simulink model "Example_OB_Dynamic_Undirected_LeaderFollower"  (R2023b)
settings: Solver=FixedStepAuto  StartTime=0.0  StopTime=20  FixedStep=0.001  RelTol=1e-3  EnableMultiTasking=on
values from neighbouring files (symbols this model uses):
  A = [0  1  0 ... (first row only)    [Code_OB_Dynamic_Undirected_LeaderFollower.m]
  ADJ = [0  1  1  0  0  0  0 ... (first row only)    [Code_OB_Dynamic_Undirected_LeaderFollower.m]
  BB = [1  0  1  0  0  1  0]*0    [Code_OB_Dynamic_Undirected_LeaderFollower.m]
  Bu = [0;0;1]    [Code_OB_Dynamic_Undirected_LeaderFollower.m]
  c = 1/lambda1    [Code_OB_Dynamic_Undirected_LeaderFollower.m]
  Cy = [1 0 0]    [Code_OB_Dynamic_Undirected_LeaderFollower.m]
  delta = 0.9*min(min(abs(eig(Q)))/max(abs(eig(P))),min(alpha))    [Code_OB_Dynamic_Undirected_LeaderFollower.m]
  eta1 = 1    [Code_OB_Dynamic_Undirected_LeaderFollower.m]
  eta2 = 1    [Code_OB_Dynamic_Undirected_LeaderFollower.m]
  eta3 = 1    [Code_OB_Dynamic_Undirected_LeaderFollower.m]
  eta4 = 1    [Code_OB_Dynamic_Undirected_LeaderFollower.m]
  eta5 = 1    [Code_OB_Dynamic_Undirected_LeaderFollower.m]
  eta6 = 1    [Code_OB_Dynamic_Undirected_LeaderFollower.m]
  F = -P*Cy'    [Code_OB_Dynamic_Undirected_LeaderFollower.m]
  K = -Bu'*P    [Code_OB_Dynamic_Undirected_LeaderFollower.m]
  kappa = 0.1    [Code_OB_Dynamic_Undirected_LeaderFollower.m]
  LL = diag(sum(ADJ,2))-ADJ    [Code_OB_Dynamic_Undirected_LeaderFollower.m]
  mu = 0.5    [Code_OB_Dynamic_Undirected_LeaderFollower.m]
  N = length(LL)    [Code_OB_Dynamic_Undirected_LeaderFollower.m]
  nr = nx    [Code_OB_Dynamic_Undirected_LeaderFollower.m]
  nx = size(A,1)    [Code_OB_Dynamic_Undirected_LeaderFollower.m]
  ny = size(Cy,1)    [Code_OB_Dynamic_Undirected_LeaderFollower.m]
  Tc = linspace(0.1,0.7,7)    [Code_OB_Dynamic_Undirected_LeaderFollower.m]
  Th = 10    [Code_OB_Dynamic_Undirected_LeaderFollower.m]
  x0 = x_leader.Data    [Code_OB_Dynamic_Undirected_LeaderFollower.m]
  x0_leader = [1 1 1]    [Code_OB_Dynamic_Undirected_LeaderFollower.m]
undefined symbols (not defined in the file or in its folder): Kri_m_Krj_1, Kri_m_Krj_2, Kri_m_Krj_3, Kri_m_Krj_4, Kri_m_Krj_5, Kri_m_Krj_6, Kri_m_Krj_7, ty0_1, ty0_2, ty0_3, ty0_4, ty0_5, ty0_6, ty0_7
settings Model: PauseTimes=0.9999  Creator=Xianwei  LastModifiedBy=30970
settings SolverCC: AlgebraicLoopSolver=LineSearch
settings DataIOCC: LimitDataPoints=on  ReturnWorkspaceOutputs=off
settings OptimizationCC: LifeSpan=inf
settings DebuggingCC: UnconnectedInputMsg=warning  UnconnectedOutputMsg=warning  UnconnectedLineMsg=warning  AllowSymbolicDim=off  SFUnexpectedBacktrackingDiag=warning  SFNoUnconditionalDefaultTransitionDiag=warning  SFExecutionAtInitializationDiag=none  ArithmeticOperatorsInVariantConditions=warning
settings ModelReferenceCC: EnableRefExpFcnMdlSchedulingChecks=on  PropagateSignalLabelsOutOfModel=off
settings SFSimCC: SimUseLocalCustomCode=off  CustomCodeUndefinedFunction=UseInterfaceOnly
settings RTWCC: RTWUseLocalCustomCode=off  DLArmComputeVersion=19.05
settings CodeAppCC: StateflowObjectComments=on
settings GRTTargetCC: TargetLangStandard=C89/C90 (ANSI)
settings ConfigComp: CovMetricSettings=dw  CovSaveCumulativeToWorkspaceVar=on  CovSaveSingleToWorkspaceVar=on  CovExternalEMLEnable=off

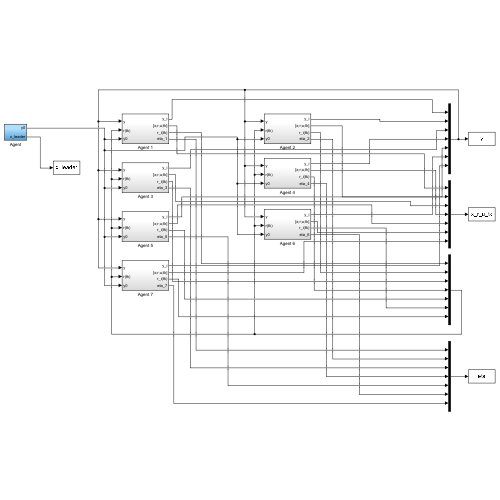
[thumbnail: Simulink's stored preview of the top-level diagram]
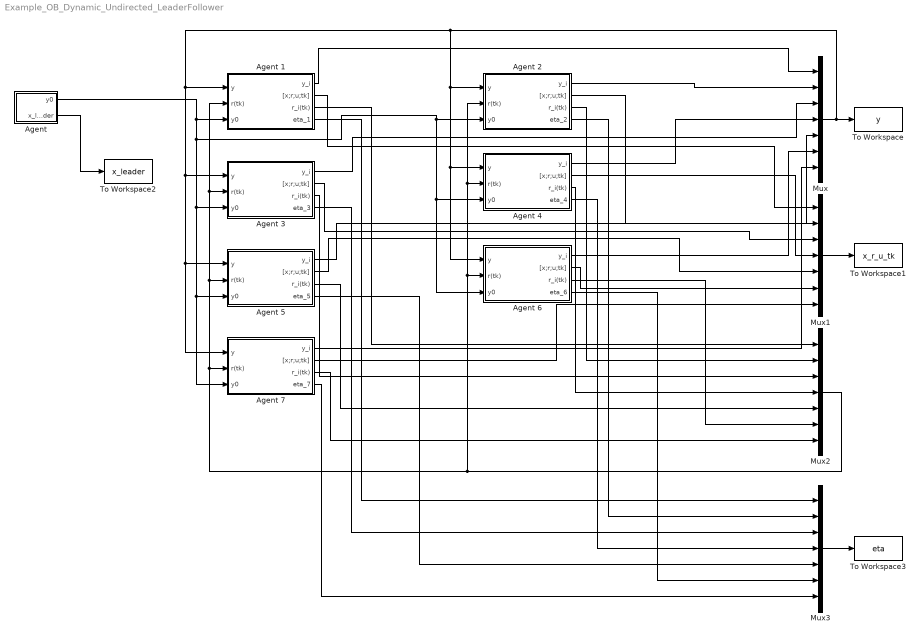
== system Example_OB_Dynamic_Undirected_LeaderFollower ==
  Agent : Subsystem
  Agent 1 : Subsystem
  Agent 2 : Subsystem
  Agent 3 : Subsystem
  Agent 4 : Subsystem
  Agent 5 : Subsystem
  Agent 6 : Subsystem
  Agent 7 : Subsystem
  Mux{,1..3} (4 alike) : Mux  Inputs=7
  To Workspace : ToWorkspace  VariableName=y  SaveFormat=Timeseries  SampleTime=-1
  To Workspace1 : ToWorkspace  VariableName=x_r_u_tk  SaveFormat=Timeseries  SampleTime=-1
  To Workspace2 : ToWorkspace  VariableName=x_leader  SaveFormat=Timeseries  SampleTime=-1
  To Workspace3 : ToWorkspace  VariableName=eta  SaveFormat=Timeseries  SampleTime=-1
  wires:
  Mux1/1 -> To Workspace1/1
  Agent 1/1(y_i) -> Mux/1
  Agent 2/1(y_i) -> Mux/2
  Agent 3/1(y_i) -> Mux/3
  Agent 4/1(y_i) -> Mux/4
  Agent 5/1(y_i) -> Mux/5
  Agent 1/2("[x;r;u;tk]") -> Mux1/1
  Agent 2/2("[x;r;u;tk]") -> Mux1/2
  Agent 3/2("[x;r;u;tk]") -> Mux1/3
  Agent 4/2("[x;r;u;tk]") -> Mux1/4
  Agent 5/2("[x;r;u;tk]") -> Mux1/5
  Agent 1/3(r_i(tk)) -> Mux2/1
  Agent 2/3(r_i(tk)) -> Mux2/2
  Agent 3/3(r_i(tk)) -> Mux2/3
  Agent 4/3(r_i(tk)) -> Mux2/4
  Agent 5/3(r_i(tk)) -> Mux2/5
  Agent 6/3(r_i(tk)) -> Mux2/6
  Agent 6/1(y_i) -> Mux/6
  Agent 6/2("[x;r;u;tk]") -> Mux1/6
  Agent 7/1(y_i) -> Mux/7
  Agent 7/2("[x;r;u;tk]") -> Mux1/7
  Agent 7/3(r_i(tk)) -> Mux2/7
  Mux/1 -> Agent 7/1(y), Agent 5/1(y), Agent 3/1(y), Agent 1/1(y), Agent 6/1(y), Agent 4/1(y), Agent 2/1(y), To Workspace/1
  Mux2/1 -> Agent 1/2(r(tk)), Agent 3/2(r(tk)), Agent 5/2(r(tk)), Agent 7/2(r(tk)), Agent 2/2(r(tk)), Agent 4/2(r(tk)), Agent 6/2(r(tk))
  Agent/1(y0) -> Agent 6/3(y0), Agent 4/3(y0), Agent 2/3(y0), Agent 7/3(y0), Agent 5/3(y0), Agent 3/3(y0), Agent 1/3(y0)
  Agent/2(x_leader) -> To Workspace2/1
  Agent 1/4(eta_1) -> Mux3/1
  Mux3/1 -> To Workspace3/1
  Agent 2/4(eta_2) -> Mux3/2
  Agent 3/4(eta_3) -> Mux3/3
  Agent 4/4(eta_4) -> Mux3/4
  Agent 5/4(eta_5) -> Mux3/5
  Agent 6/4(eta_6) -> Mux3/6
  Agent 7/4(eta_7) -> Mux3/7

== system Example_OB_Dynamic_Undirected_LeaderFollower/Agent ==
  A : Gain  Gain=A  Multiplication=Matrix(K*u)
  Cy : Gain  Gain=Cy  Multiplication=Matrix(K*u)
  Integrator : Integrator  InitialCondition=x0_leader  ContinuousStateAttributes='x1'
  y0 : Outport
  x_leader : Outport  Port=2
  wires:
  Integrator/1 -> x_leader/1, A/1, Cy/1
  A/1 -> Integrator/1
  Cy/1 -> y0/1

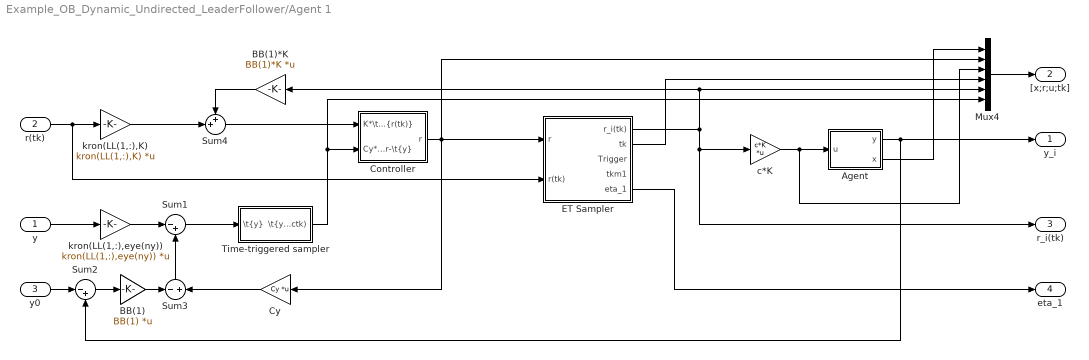
== system Example_OB_Dynamic_Undirected_LeaderFollower/Agent 1 ==
  y : Inport
  r(tk) : Inport  Port=2
  y0 : Inport  Port=3
  Agent : Subsystem
  BB(1) : Gain  Gain=BB(1)  Multiplication=Matrix(K*u)
  BB(1)*K : Gain  Gain=BB(1)*K  Multiplication=Matrix(K*u)
  Controller : Subsystem
  Cy : Gain  Gain=Cy  Multiplication=Matrix(K*u)
  ET Sampler : Subsystem
  Mux4 : Mux  Inputs=6
  Sum1 : Sum  Inputs=|-+
  Sum2 : Sum  Inputs=|-+
  Sum3 : Sum  Inputs=-|+
  Sum4 : Sum  Inputs=++|
  Time-triggered sampler : Subsystem
  c*K : Gain  Gain=c*K  Multiplication=Matrix(K*u)
  kron(LL(1,:),K) : Gain  Gain=kron(LL(1,:),K)  Multiplication=Matrix(K*u)
  kron(LL(1,:),eye(ny)) : Gain  Gain=kron(LL(1,:),eye(ny))  Multiplication=Matrix(K*u)
  y_i : Outport
  "[x;r;u;tk]" : Outport  Port=2
  r_i(tk) : Outport  Port=3
  eta_1 : Outport  Port=4
  wires:
  Agent/2(x) -> Mux4/1
  Mux4/1 -> "[x;r;u;tk]"/1
  ET Sampler/2(tk) -> Mux4/4
  c*K/1 -> Agent/1(u), Mux4/3
  y/1 -> kron(LL(1,:),eye(ny))/1
  r(tk)/1 -> kron(LL(1,:),K)/1, ET Sampler/2(r(tk))
  kron(LL(1,:),K)/1 -> Sum4/2
  ET Sampler/1(r_i(tk)) -> BB(1)*K/1, Mux4/5, c*K/1, r_i(tk)/1
  Controller/1(r) -> Cy/1, ET Sampler/1(r), Mux4/2
  Cy/1 -> Sum3/2
  Sum1/1 -> Time-triggered sampler/1("\\t{y}")
  kron(LL(1,:),eye(ny))/1 -> Sum1/1
  Time-triggered sampler/1("\\t{y}(ctk)") -> Mux4/6, Controller/2("Cy*r-\\t{y}")
  y0/1 -> Sum2/1
  Agent/1(y) -> Sum2/2, y_i/1
  Sum2/1 -> BB(1)/1
  BB(1)/1 -> Sum3/1
  Sum3/1 -> Sum1/2
  BB(1)*K/1 -> Sum4/1
  Sum4/1 -> Controller/1("K*\\t{r(tk)}")
  ET Sampler/5(eta_1) -> eta_1/1

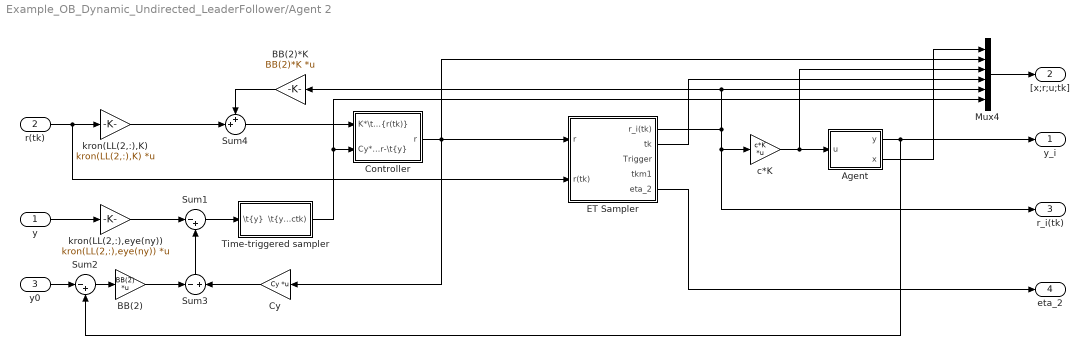
== system Example_OB_Dynamic_Undirected_LeaderFollower/Agent 2 ==
  y : Inport
  r(tk) : Inport  Port=2
  y0 : Inport  Port=3
  Agent : Subsystem
  BB(2) : Gain  Gain=BB(2)  Multiplication=Matrix(K*u)
  BB(2)*K : Gain  Gain=BB(2)*K  Multiplication=Matrix(K*u)
  Controller : Subsystem
  Cy : Gain  Gain=Cy  Multiplication=Matrix(K*u)
  ET Sampler : Subsystem
  Mux4 : Mux  Inputs=6
  Sum1 : Sum  Inputs=|-+
  Sum2 : Sum  Inputs=|-+
  Sum3 : Sum  Inputs=-|+
  Sum4 : Sum  Inputs=++|
  Time-triggered sampler : Subsystem
  c*K : Gain  Gain=c*K  Multiplication=Matrix(K*u)
  kron(LL(2,:),K) : Gain  Gain=kron(LL(2,:),K)  Multiplication=Matrix(K*u)
  kron(LL(2,:),eye(ny)) : Gain  Gain=kron(LL(2,:),eye(ny))  Multiplication=Matrix(K*u)
  y_i : Outport
  "[x;r;u;tk]" : Outport  Port=2
  r_i(tk) : Outport  Port=3
  eta_2 : Outport  Port=4
  wires:
  c*K/1 -> Agent/1(u), Mux4/3
  r(tk)/1 -> ET Sampler/2(r(tk)), kron(LL(2,:),K)/1
  kron(LL(2,:),K)/1 -> Sum4/2
  Mux4/1 -> "[x;r;u;tk]"/1
  Controller/1(r) -> ET Sampler/1(r), Mux4/2, Cy/1
  Agent/2(x) -> Mux4/1
  kron(LL(2,:),eye(ny))/1 -> Sum1/1
  ET Sampler/2(tk) -> Mux4/4
  y/1 -> kron(LL(2,:),eye(ny))/1
  Cy/1 -> Sum3/2
  Sum1/1 -> Time-triggered sampler/1("\\t{y}")
  Time-triggered sampler/1("\\t{y}(ctk)") -> Mux4/6, Controller/2("Cy*r-\\t{y}")
  y0/1 -> Sum2/1
  Agent/1(y) -> Sum2/2, y_i/1
  BB(2)/1 -> Sum3/1
  Sum2/1 -> BB(2)/1
  Sum3/1 -> Sum1/2
  BB(2)*K/1 -> Sum4/1
  ET Sampler/1(r_i(tk)) -> BB(2)*K/1, Mux4/5, r_i(tk)/1, c*K/1
  Sum4/1 -> Controller/1("K*\\t{r(tk)}")
  ET Sampler/5(eta_2) -> eta_2/1

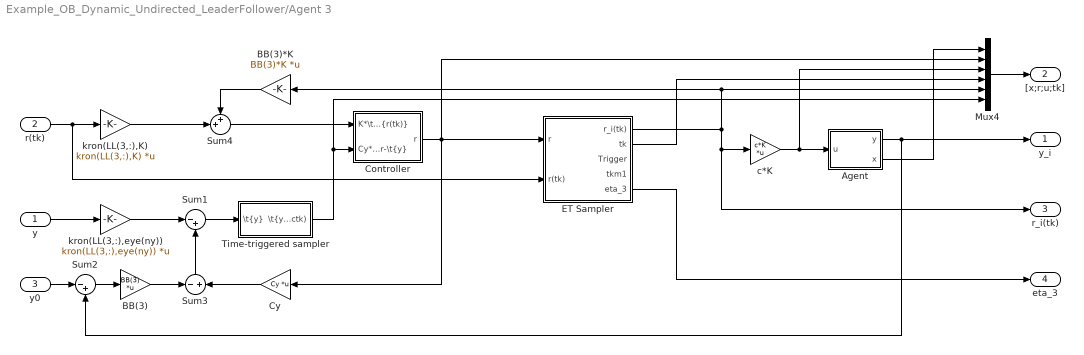
== system Example_OB_Dynamic_Undirected_LeaderFollower/Agent 3 ==
  y : Inport
  r(tk) : Inport  Port=2
  y0 : Inport  Port=3
  Agent : Subsystem
  BB(3) : Gain  Gain=BB(3)  Multiplication=Matrix(K*u)
  BB(3)*K : Gain  Gain=BB(3)*K  Multiplication=Matrix(K*u)
  Controller : Subsystem
  Cy : Gain  Gain=Cy  Multiplication=Matrix(K*u)
  ET Sampler : Subsystem
  Mux4 : Mux  Inputs=6
  Sum1 : Sum  Inputs=|-+
  Sum2 : Sum  Inputs=|-+
  Sum3 : Sum  Inputs=-|+
  Sum4 : Sum  Inputs=++|
  Time-triggered sampler : Subsystem
  c*K : Gain  Gain=c*K  Multiplication=Matrix(K*u)
  kron(LL(3,:),K) : Gain  Gain=kron(LL(3,:),K)  Multiplication=Matrix(K*u)
  kron(LL(3,:),eye(ny)) : Gain  Gain=kron(LL(3,:),eye(ny))  Multiplication=Matrix(K*u)
  y_i : Outport
  "[x;r;u;tk]" : Outport  Port=2
  r_i(tk) : Outport  Port=3
  eta_3 : Outport  Port=4
  wires:
  c*K/1 -> Agent/1(u), Mux4/3
  r(tk)/1 -> ET Sampler/2(r(tk)), kron(LL(3,:),K)/1
  kron(LL(3,:),K)/1 -> Sum4/2
  Mux4/1 -> "[x;r;u;tk]"/1
  Controller/1(r) -> ET Sampler/1(r), Mux4/2, Cy/1
  Agent/2(x) -> Mux4/1
  kron(LL(3,:),eye(ny))/1 -> Sum1/1
  ET Sampler/2(tk) -> Mux4/4
  y/1 -> kron(LL(3,:),eye(ny))/1
  Cy/1 -> Sum3/2
  Sum1/1 -> Time-triggered sampler/1("\\t{y}")
  Time-triggered sampler/1("\\t{y}(ctk)") -> Mux4/6, Controller/2("Cy*r-\\t{y}")
  Sum2/1 -> BB(3)/1
  BB(3)/1 -> Sum3/1
  Agent/1(y) -> Sum2/2, y_i/1
  y0/1 -> Sum2/1
  Sum3/1 -> Sum1/2
  BB(3)*K/1 -> Sum4/1
  ET Sampler/1(r_i(tk)) -> BB(3)*K/1, Mux4/5, r_i(tk)/1, c*K/1
  Sum4/1 -> Controller/1("K*\\t{r(tk)}")
  ET Sampler/5(eta_3) -> eta_3/1

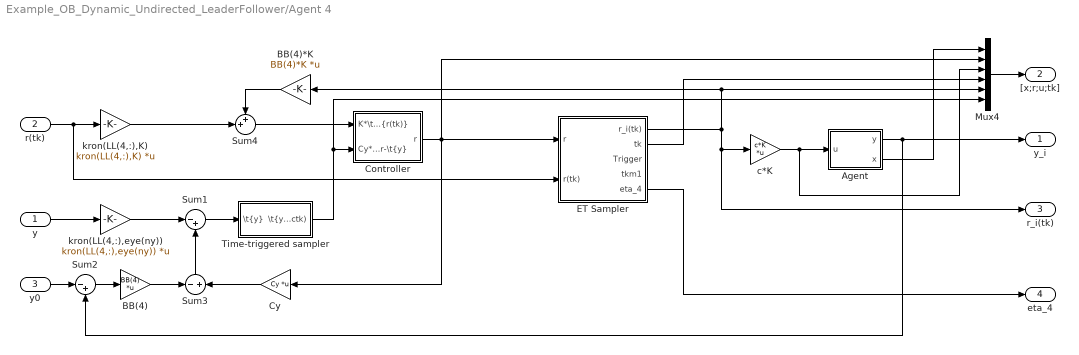
== system Example_OB_Dynamic_Undirected_LeaderFollower/Agent 4 ==
  y : Inport
  r(tk) : Inport  Port=2
  y0 : Inport  Port=3
  Agent : Subsystem
  BB(4) : Gain  Gain=BB(4)  Multiplication=Matrix(K*u)
  BB(4)*K : Gain  Gain=BB(4)*K  Multiplication=Matrix(K*u)
  Controller : Subsystem
  Cy : Gain  Gain=Cy  Multiplication=Matrix(K*u)
  ET Sampler : Subsystem
  Mux4 : Mux  Inputs=6
  Sum1 : Sum  Inputs=|-+
  Sum2 : Sum  Inputs=|-+
  Sum3 : Sum  Inputs=-|+
  Sum4 : Sum  Inputs=++|
  Time-triggered sampler : Subsystem
  c*K : Gain  Gain=c*K  Multiplication=Matrix(K*u)
  kron(LL(4,:),K) : Gain  Gain=kron(LL(4,:),K)  Multiplication=Matrix(K*u)
  kron(LL(4,:),eye(ny)) : Gain  Gain=kron(LL(4,:),eye(ny))  Multiplication=Matrix(K*u)
  y_i : Outport
  "[x;r;u;tk]" : Outport  Port=2
  r_i(tk) : Outport  Port=3
  eta_4 : Outport  Port=4
  wires:
  y/1 -> kron(LL(4,:),eye(ny))/1
  Sum1/1 -> Time-triggered sampler/1("\\t{y}")
  Mux4/1 -> "[x;r;u;tk]"/1
  c*K/1 -> Agent/1(u), Mux4/3
  ET Sampler/2(tk) -> Mux4/4
  r(tk)/1 -> ET Sampler/2(r(tk)), kron(LL(4,:),K)/1
  Controller/1(r) -> ET Sampler/1(r), Mux4/2, Cy/1
  Agent/2(x) -> Mux4/1
  kron(LL(4,:),K)/1 -> Sum4/2
  kron(LL(4,:),eye(ny))/1 -> Sum1/1
  Time-triggered sampler/1("\\t{y}(ctk)") -> Mux4/6, Controller/2("Cy*r-\\t{y}")
  Sum2/1 -> BB(4)/1
  BB(4)/1 -> Sum3/1
  Agent/1(y) -> Sum2/2, y_i/1
  y0/1 -> Sum2/1
  Sum3/1 -> Sum1/2
  Cy/1 -> Sum3/2
  BB(4)*K/1 -> Sum4/1
  ET Sampler/1(r_i(tk)) -> BB(4)*K/1, Mux4/5, r_i(tk)/1, c*K/1
  Sum4/1 -> Controller/1("K*\\t{r(tk)}")
  ET Sampler/5(eta_4) -> eta_4/1

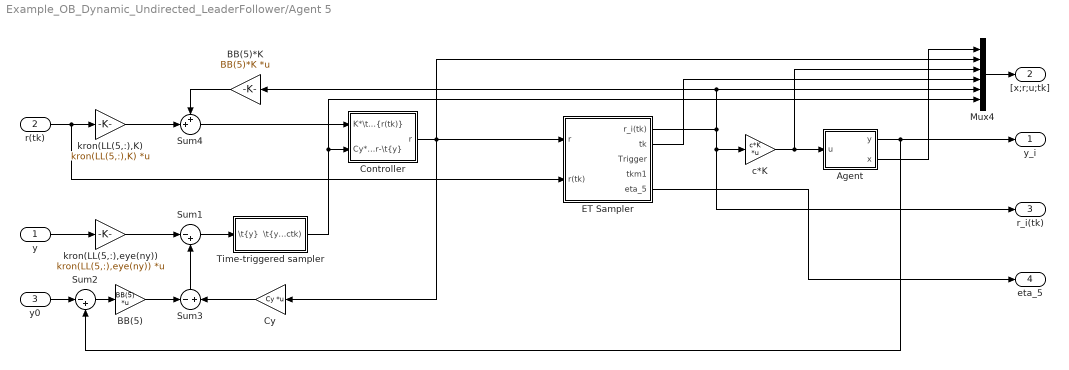
== system Example_OB_Dynamic_Undirected_LeaderFollower/Agent 5 ==
  y : Inport
  r(tk) : Inport  Port=2
  y0 : Inport  Port=3
  Agent : Subsystem
  BB(5) : Gain  Gain=BB(5)  Multiplication=Matrix(K*u)
  BB(5)*K : Gain  Gain=BB(5)*K  Multiplication=Matrix(K*u)
  Controller : Subsystem
  Cy : Gain  Gain=Cy  Multiplication=Matrix(K*u)
  ET Sampler : Subsystem
  Mux4 : Mux  Inputs=6
  Sum1 : Sum  Inputs=|-+
  Sum2 : Sum  Inputs=|-+
  Sum3 : Sum  Inputs=-|+
  Sum4 : Sum  Inputs=++|
  Time-triggered sampler : Subsystem
  c*K : Gain  Gain=c*K  Multiplication=Matrix(K*u)
  kron(LL(5,:),K) : Gain  Gain=kron(LL(5,:),K)  Multiplication=Matrix(K*u)
  kron(LL(5,:),eye(ny)) : Gain  Gain=kron(LL(5,:),eye(ny))  Multiplication=Matrix(K*u)
  y_i : Outport
  "[x;r;u;tk]" : Outport  Port=2
  r_i(tk) : Outport  Port=3
  eta_5 : Outport  Port=4
  wires:
  kron(LL(5,:),eye(ny))/1 -> Sum1/1
  kron(LL(5,:),K)/1 -> Sum4/2
  Agent/2(x) -> Mux4/1
  Controller/1(r) -> ET Sampler/1(r), Mux4/2, Cy/1
  ET Sampler/2(tk) -> Mux4/4
  Sum1/1 -> Time-triggered sampler/1("\\t{y}")
  c*K/1 -> Agent/1(u), Mux4/3
  Mux4/1 -> "[x;r;u;tk]"/1
  r(tk)/1 -> ET Sampler/2(r(tk)), kron(LL(5,:),K)/1
  y/1 -> kron(LL(5,:),eye(ny))/1
  Time-triggered sampler/1("\\t{y}(ctk)") -> Mux4/6, Controller/2("Cy*r-\\t{y}")
  Sum2/1 -> BB(5)/1
  BB(5)/1 -> Sum3/1
  Agent/1(y) -> Sum2/2, y_i/1
  y0/1 -> Sum2/1
  Cy/1 -> Sum3/2
  Sum3/1 -> Sum1/2
  BB(5)*K/1 -> Sum4/1
  ET Sampler/1(r_i(tk)) -> Mux4/5, BB(5)*K/1, r_i(tk)/1, c*K/1
  Sum4/1 -> Controller/1("K*\\t{r(tk)}")
  ET Sampler/5(eta_5) -> eta_5/1

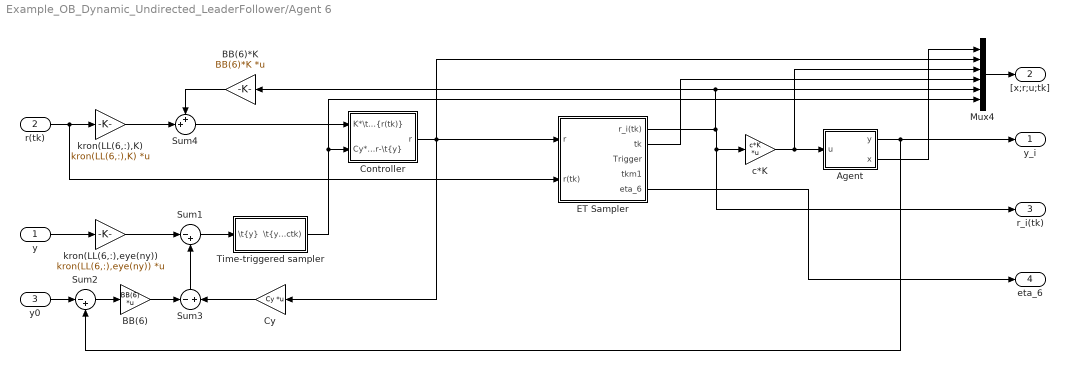
== system Example_OB_Dynamic_Undirected_LeaderFollower/Agent 6 ==
  y : Inport
  r(tk) : Inport  Port=2
  y0 : Inport  Port=3
  Agent : Subsystem
  BB(6) : Gain  Gain=BB(6)  Multiplication=Matrix(K*u)
  BB(6)*K : Gain  Gain=BB(6)*K  Multiplication=Matrix(K*u)
  Controller : Subsystem
  Cy : Gain  Gain=Cy  Multiplication=Matrix(K*u)
  ET Sampler : Subsystem
  Mux4 : Mux  Inputs=6
  Sum1 : Sum  Inputs=|-+
  Sum2 : Sum  Inputs=|-+
  Sum3 : Sum  Inputs=-|+
  Sum4 : Sum  Inputs=++|
  Time-triggered sampler : Subsystem
  c*K : Gain  Gain=c*K  Multiplication=Matrix(K*u)
  kron(LL(6,:),K) : Gain  Gain=kron(LL(6,:),K)  Multiplication=Matrix(K*u)
  kron(LL(6,:),eye(ny)) : Gain  Gain=kron(LL(6,:),eye(ny))  Multiplication=Matrix(K*u)
  y_i : Outport
  "[x;r;u;tk]" : Outport  Port=2
  r_i(tk) : Outport  Port=3
  eta_6 : Outport  Port=4
  wires:
  r(tk)/1 -> ET Sampler/2(r(tk)), kron(LL(6,:),K)/1
  Sum1/1 -> Time-triggered sampler/1("\\t{y}")
  c*K/1 -> Agent/1(u), Mux4/3
  ET Sampler/2(tk) -> Mux4/4
  Controller/1(r) -> ET Sampler/1(r), Mux4/2, Cy/1
  Agent/2(x) -> Mux4/1
  Mux4/1 -> "[x;r;u;tk]"/1
  kron(LL(6,:),eye(ny))/1 -> Sum1/1
  y/1 -> kron(LL(6,:),eye(ny))/1
  kron(LL(6,:),K)/1 -> Sum4/2
  Time-triggered sampler/1("\\t{y}(ctk)") -> Mux4/6, Controller/2("Cy*r-\\t{y}")
  Sum2/1 -> BB(6)/1
  BB(6)/1 -> Sum3/1
  Agent/1(y) -> Sum2/2, y_i/1
  y0/1 -> Sum2/1
  Cy/1 -> Sum3/2
  Sum3/1 -> Sum1/2
  BB(6)*K/1 -> Sum4/1
  ET Sampler/1(r_i(tk)) -> Mux4/5, BB(6)*K/1, r_i(tk)/1, c*K/1
  Sum4/1 -> Controller/1("K*\\t{r(tk)}")
  ET Sampler/5(eta_6) -> eta_6/1

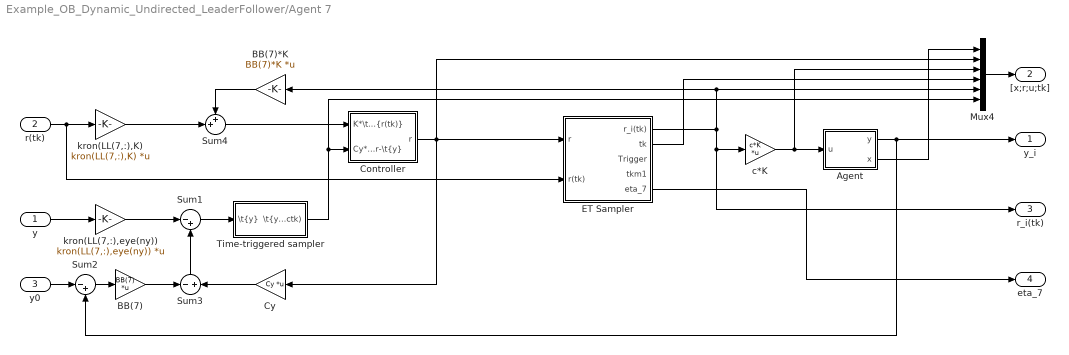
== system Example_OB_Dynamic_Undirected_LeaderFollower/Agent 7 ==
  y : Inport
  r(tk) : Inport  Port=2
  y0 : Inport  Port=3
  Agent : Subsystem
  BB(7) : Gain  Gain=BB(7)  Multiplication=Matrix(K*u)
  BB(7)*K : Gain  Gain=BB(7)*K  Multiplication=Matrix(K*u)
  Controller : Subsystem
  Cy : Gain  Gain=Cy  Multiplication=Matrix(K*u)
  ET Sampler : Subsystem
  Mux4 : Mux  Inputs=6
  Sum1 : Sum  Inputs=|-+
  Sum2 : Sum  Inputs=|-+
  Sum3 : Sum  Inputs=-|+
  Sum4 : Sum  Inputs=++|
  Time-triggered sampler : Subsystem
  c*K : Gain  Gain=c*K  Multiplication=Matrix(K*u)
  kron(LL(7,:),K) : Gain  Gain=kron(LL(7,:),K)  Multiplication=Matrix(K*u)
  kron(LL(7,:),eye(ny)) : Gain  Gain=kron(LL(7,:),eye(ny))  Multiplication=Matrix(K*u)
  y_i : Outport
  "[x;r;u;tk]" : Outport  Port=2
  r_i(tk) : Outport  Port=3
  eta_7 : Outport  Port=4
  wires:
  y/1 -> kron(LL(7,:),eye(ny))/1
  kron(LL(7,:),K)/1 -> Sum4/2
  Agent/2(x) -> Mux4/1
  Controller/1(r) -> ET Sampler/1(r), Mux4/2, Cy/1
  kron(LL(7,:),eye(ny))/1 -> Sum1/1
  r(tk)/1 -> kron(LL(7,:),K)/1, ET Sampler/2(r(tk))
  c*K/1 -> Agent/1(u), Mux4/3
  ET Sampler/2(tk) -> Mux4/4
  Sum1/1 -> Time-triggered sampler/1("\\t{y}")
  Mux4/1 -> "[x;r;u;tk]"/1
  Time-triggered sampler/1("\\t{y}(ctk)") -> Mux4/6, Controller/2("Cy*r-\\t{y}")
  Sum2/1 -> BB(7)/1
  BB(7)/1 -> Sum3/1
  Agent/1(y) -> Sum2/2, y_i/1
  y0/1 -> Sum2/1
  Cy/1 -> Sum3/2
  Sum3/1 -> Sum1/2
  BB(7)*K/1 -> Sum4/1
  ET Sampler/1(r_i(tk)) -> BB(7)*K/1, Mux4/5, r_i(tk)/1, c*K/1
  Sum4/1 -> Controller/1("K*\\t{r(tk)}")
  ET Sampler/5(eta_7) -> eta_7/1

== system Example_OB_Dynamic_Undirected_LeaderFollower/Agent 1/Agent ==
  u : Inport
  A : Gain  Gain=A  Multiplication=Matrix(K*u)
  Bu : Gain  Gain=Bu  Multiplication=Matrix(K*u)
  Cy : Gain  Gain=Cy  Multiplication=Matrix(K*u)
  Integrator : Integrator  InitialCondition=x0(1:nx)  ContinuousStateAttributes='x1'
  Sum5 : Sum  Inputs=|++
  y : Outport
  x : Outport  Port=2
  wires:
  Integrator/1 -> x/1, A/1, Cy/1
  A/1 -> Sum5/2
  Sum5/1 -> Integrator/1
  u/1 -> Bu/1
  Bu/1 -> Sum5/1
  Cy/1 -> y/1

== system Example_OB_Dynamic_Undirected_LeaderFollower/Agent 1/Controller ==
  "K*\\t{r(tk)}" : Inport
  "Cy*r-\\t{y}" : Inport  Port=2
  A : Gain  Gain=A  Multiplication=Matrix(K*u)
  Bu : Gain  Gain=Bu  Multiplication=Matrix(K*u)
  F : Gain  Gain=F  Multiplication=Matrix(K*u)
  Integrator : Integrator  InitialCondition=zeros(nr,1)  ContinuousStateAttributes='r1'
  Sum5 : Sum  Inputs=+++
  c : Gain  Gain=c  Multiplication=Matrix(K*u)
  r : Outport
  wires:
  A/1 -> Sum5/3
  Sum5/1 -> Integrator/1
  Integrator/1 -> r/1, A/1
  "K*\\t{r(tk)}"/1 -> c/1
  Bu/1 -> Sum5/1
  "Cy*r-\\t{y}"/1 -> F/1
  F/1 -> Sum5/2
  c/1 -> Bu/1

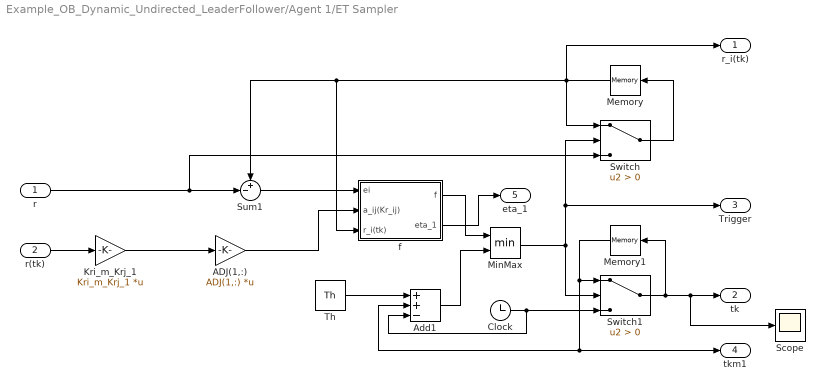
== system Example_OB_Dynamic_Undirected_LeaderFollower/Agent 1/ET Sampler ==
  r : Inport
  r(tk) : Inport  Port=2
  ADJ(1,:) : Gain  Gain=ADJ(1,:)  Multiplication=Matrix(K*u)
  Add1 : Sum  Inputs=++-
  Clock : Clock
  Kri_m_Krj_1 : Gain  Gain=Kri_m_Krj_1  Multiplication=Matrix(K*u)
  Memory : Memory  InitialCondition=zeros(nr,1)  StateName=tilde_x
  Memory1 : Memory  StateName=tilde_x
  MinMax : MinMax  Inputs=2
  Scope : Scope
  Sum1 : Sum  Inputs=+-|
  Switch : Switch  Criteria=u2 > Threshold  SaturateOnIntegerOverflow=off  InputSameDT=off
  Switch1 : Switch  Criteria=u2 > Threshold  SaturateOnIntegerOverflow=off  InputSameDT=off
  Th : Constant  Value=Th
  f : Subsystem
  r_i(tk) : Outport
  tk : Outport  Port=2
  Trigger : Outport  Port=3
  tkm1 : Outport  Port=4
  eta_1 : Outport  Port=5
  wires:
  Clock/1 -> Add1/3, Switch1/3
  Memory1/1 -> Switch1/1, Add1/2, tkm1/1
  Switch1/1 -> Scope/1, tk/1, Memory1/1
  Switch/1 -> Memory/1
  Sum1/1 -> f/1(ei)
  Memory/1 -> f/3(r_i(tk)), Sum1/1, r_i(tk)/1, Switch/1
  Kri_m_Krj_1/1 -> ADJ(1,:)/1
  r/1 -> Sum1/2, Switch/3
  r(tk)/1 -> Kri_m_Krj_1/1
  ADJ(1,:)/1 -> f/2(a_ij(Kr_ij))
  Th/1 -> Add1/1
  f/1(f) -> MinMax/1
  MinMax/1 -> Switch1/2, Trigger/1, Switch/2
  Add1/1 -> MinMax/2
  f/2(eta_1) -> eta_1/1

== system Example_OB_Dynamic_Undirected_LeaderFollower/Agent 1/Time-triggered sampler ==
  note: mod函数需要Tc的精度与仿真步长的精度一致，否则不能正确运算
  "\\t{y}" : Inport
  Clock : Clock
  Math Function : Math  Operator=mod
  Memory : Memory  InitialCondition=ty0_1  StateName=tilde_x
  Scope : Scope
  Switch : Switch  Criteria=u2 > Threshold  SaturateOnIntegerOverflow=off  InputSameDT=off
  Tc : Constant  Value=Tc(1)
  "\\t{y}(ctk)" : Outport
  wires:
  Switch/1 -> "\\t{y}(ctk)"/1, Memory/1
  "\\t{y}"/1 -> Switch/3
  Memory/1 -> Switch/1
  Tc/1 -> Math Function/2
  Clock/1 -> Math Function/1
  Math Function/1 -> Scope/1, Switch/2

== system Example_OB_Dynamic_Undirected_LeaderFollower/Agent 2/Agent ==
  u : Inport
  A : Gain  Gain=A  Multiplication=Matrix(K*u)
  Bu : Gain  Gain=Bu  Multiplication=Matrix(K*u)
  Cy : Gain  Gain=Cy  Multiplication=Matrix(K*u)
  Integrator : Integrator  InitialCondition=x0(nx+1:2*nx)  ContinuousStateAttributes='x1'
  Sum5 : Sum  Inputs=|++
  y : Outport
  x : Outport  Port=2
  wires:
  Integrator/1 -> x/1, A/1, Cy/1
  A/1 -> Sum5/2
  Sum5/1 -> Integrator/1
  u/1 -> Bu/1
  Bu/1 -> Sum5/1
  Cy/1 -> y/1

== system Example_OB_Dynamic_Undirected_LeaderFollower/Agent 2/Controller ==
  "K*\\t{r(tk)}" : Inport
  "Cy*r-\\t{y}" : Inport  Port=2
  A : Gain  Gain=A  Multiplication=Matrix(K*u)
  Bu : Gain  Gain=Bu  Multiplication=Matrix(K*u)
  F : Gain  Gain=F  Multiplication=Matrix(K*u)
  Integrator : Integrator  InitialCondition=zeros(nr,1)  ContinuousStateAttributes='r1'
  Sum5 : Sum  Inputs=+++
  c : Gain  Gain=c  Multiplication=Matrix(K*u)
  r : Outport
  wires:
  A/1 -> Sum5/3
  Sum5/1 -> Integrator/1
  Integrator/1 -> r/1, A/1
  "K*\\t{r(tk)}"/1 -> c/1
  Bu/1 -> Sum5/1
  "Cy*r-\\t{y}"/1 -> F/1
  F/1 -> Sum5/2
  c/1 -> Bu/1

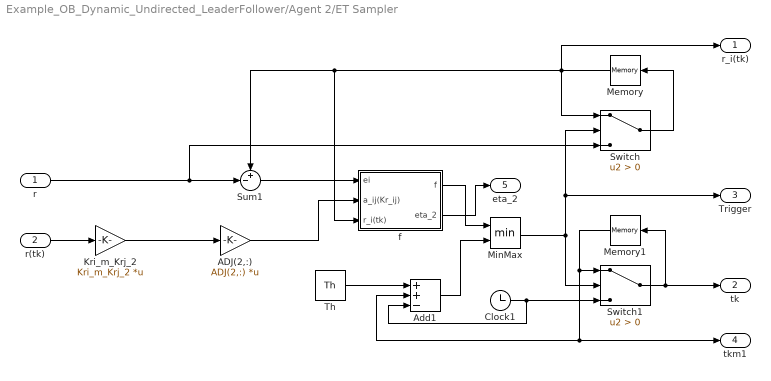
== system Example_OB_Dynamic_Undirected_LeaderFollower/Agent 2/ET Sampler ==
  r : Inport
  r(tk) : Inport  Port=2
  ADJ(2,:) : Gain  Gain=ADJ(2,:)  Multiplication=Matrix(K*u)
  Add1 : Sum  Inputs=++-
  Clock1 : Clock
  Kri_m_Krj_2 : Gain  Gain=Kri_m_Krj_2  Multiplication=Matrix(K*u)
  Memory : Memory  InitialCondition=zeros(nr,1)  StateName=tilde_x
  Memory1 : Memory  StateName=tilde_x
  MinMax : MinMax  Inputs=2
  Sum1 : Sum  Inputs=+-|
  Switch : Switch  Criteria=u2 > Threshold  SaturateOnIntegerOverflow=off  InputSameDT=off
  Switch1 : Switch  Criteria=u2 > Threshold  SaturateOnIntegerOverflow=off  InputSameDT=off
  Th : Constant  Value=Th
  f : Subsystem
  r_i(tk) : Outport
  tk : Outport  Port=2
  Trigger : Outport  Port=3
  tkm1 : Outport  Port=4
  eta_2 : Outport  Port=5
  wires:
  Switch/1 -> Memory/1
  Sum1/1 -> f/1(ei)
  r/1 -> Sum1/2, Switch/3
  Memory/1 -> r_i(tk)/1, f/3(r_i(tk)), Sum1/1, Switch/1
  r(tk)/1 -> Kri_m_Krj_2/1
  Kri_m_Krj_2/1 -> ADJ(2,:)/1
  ADJ(2,:)/1 -> f/2(a_ij(Kr_ij))
  Switch1/1 -> tk/1, Memory1/1
  MinMax/1 -> Switch1/2, Switch/2, Trigger/1
  Memory1/1 -> Switch1/1, Add1/2, tkm1/1
  Th/1 -> Add1/1
  Add1/1 -> MinMax/2
  Clock1/1 -> Switch1/3, Add1/3
  f/1(f) -> MinMax/1
  f/2(eta_2) -> eta_2/1

== system Example_OB_Dynamic_Undirected_LeaderFollower/Agent 2/Time-triggered sampler ==
  "\\t{y}" : Inport
  Clock : Clock
  Math Function : Math  Operator=mod
  Memory : Memory  InitialCondition=ty0_2  StateName=tilde_x
  Switch : Switch  Criteria=u2 > Threshold  SaturateOnIntegerOverflow=off  InputSameDT=off
  Tc : Constant  Value=Tc(2)
  "\\t{y}(ctk)" : Outport
  wires:
  Switch/1 -> "\\t{y}(ctk)"/1, Memory/1
  "\\t{y}"/1 -> Switch/3
  Memory/1 -> Switch/1
  Tc/1 -> Math Function/2
  Clock/1 -> Math Function/1
  Math Function/1 -> Switch/2

== system Example_OB_Dynamic_Undirected_LeaderFollower/Agent 3/Agent ==
  u : Inport
  A : Gain  Gain=A  Multiplication=Matrix(K*u)
  Bu : Gain  Gain=Bu  Multiplication=Matrix(K*u)
  Cy : Gain  Gain=Cy  Multiplication=Matrix(K*u)
  Integrator : Integrator  InitialCondition=x0(2*nx+1:3*nx)  ContinuousStateAttributes='x1'
  Sum5 : Sum  Inputs=|++
  y : Outport
  x : Outport  Port=2
  wires:
  Integrator/1 -> x/1, A/1, Cy/1
  A/1 -> Sum5/2
  Sum5/1 -> Integrator/1
  u/1 -> Bu/1
  Bu/1 -> Sum5/1
  Cy/1 -> y/1

== system Example_OB_Dynamic_Undirected_LeaderFollower/Agent 3/Controller ==
  "K*\\t{r(tk)}" : Inport
  "Cy*r-\\t{y}" : Inport  Port=2
  A : Gain  Gain=A  Multiplication=Matrix(K*u)
  Bu : Gain  Gain=Bu  Multiplication=Matrix(K*u)
  F : Gain  Gain=F  Multiplication=Matrix(K*u)
  Integrator : Integrator  InitialCondition=zeros(nr,1)  ContinuousStateAttributes='r1'
  Sum5 : Sum  Inputs=+++
  c : Gain  Gain=c  Multiplication=Matrix(K*u)
  r : Outport
  wires:
  A/1 -> Sum5/3
  Sum5/1 -> Integrator/1
  Integrator/1 -> r/1, A/1
  "K*\\t{r(tk)}"/1 -> c/1
  Bu/1 -> Sum5/1
  "Cy*r-\\t{y}"/1 -> F/1
  F/1 -> Sum5/2
  c/1 -> Bu/1

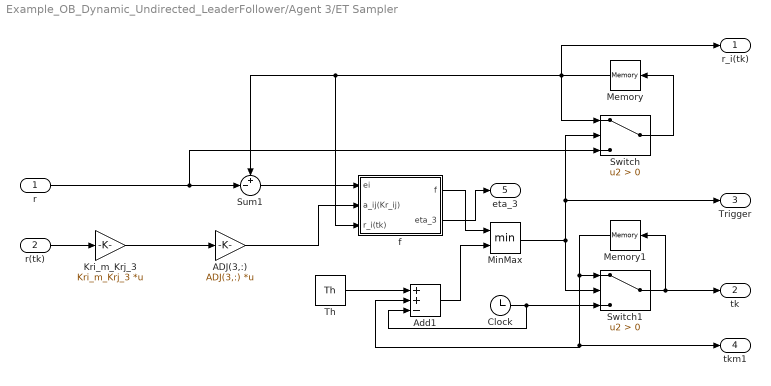
== system Example_OB_Dynamic_Undirected_LeaderFollower/Agent 3/ET Sampler ==
  r : Inport
  r(tk) : Inport  Port=2
  ADJ(3,:) : Gain  Gain=ADJ(3,:)  Multiplication=Matrix(K*u)
  Add1 : Sum  Inputs=++-
  Clock : Clock
  Kri_m_Krj_3 : Gain  Gain=Kri_m_Krj_3  Multiplication=Matrix(K*u)
  Memory : Memory  InitialCondition=zeros(nr,1)  StateName=tilde_x
  Memory1 : Memory  StateName=tilde_x
  MinMax : MinMax  Inputs=2
  Sum1 : Sum  Inputs=+-|
  Switch : Switch  Criteria=u2 > Threshold  SaturateOnIntegerOverflow=off  InputSameDT=off
  Switch1 : Switch  Criteria=u2 > Threshold  SaturateOnIntegerOverflow=off  InputSameDT=off
  Th : Constant  Value=Th
  f : Subsystem
  r_i(tk) : Outport
  tk : Outport  Port=2
  Trigger : Outport  Port=3
  tkm1 : Outport  Port=4
  eta_3 : Outport  Port=5
  wires:
  Switch/1 -> Memory/1
  Sum1/1 -> f/1(ei)
  r/1 -> Sum1/2, Switch/3
  Memory/1 -> Switch/1, r_i(tk)/1, f/3(r_i(tk)), Sum1/1
  r(tk)/1 -> Kri_m_Krj_3/1
  Kri_m_Krj_3/1 -> ADJ(3,:)/1
  ADJ(3,:)/1 -> f/2(a_ij(Kr_ij))
  Switch1/1 -> tk/1, Memory1/1
  MinMax/1 -> Switch1/2, Switch/2, Trigger/1
  Memory1/1 -> Switch1/1, Add1/2, tkm1/1
  Th/1 -> Add1/1
  Add1/1 -> MinMax/2
  Clock/1 -> Switch1/3, Add1/3
  f/1(f) -> MinMax/1
  f/2(eta_3) -> eta_3/1

== system Example_OB_Dynamic_Undirected_LeaderFollower/Agent 3/Time-triggered sampler ==
  "\\t{y}" : Inport
  Clock : Clock
  Math Function : Math  Operator=mod
  Memory : Memory  InitialCondition=ty0_3  StateName=tilde_x
  Switch : Switch  Criteria=u2 > Threshold  SaturateOnIntegerOverflow=off  InputSameDT=off
  Tc : Constant  Value=Tc(3)
  "\\t{y}(ctk)" : Outport
  wires:
  Switch/1 -> "\\t{y}(ctk)"/1, Memory/1
  "\\t{y}"/1 -> Switch/3
  Memory/1 -> Switch/1
  Tc/1 -> Math Function/2
  Clock/1 -> Math Function/1
  Math Function/1 -> Switch/2

== system Example_OB_Dynamic_Undirected_LeaderFollower/Agent 4/Agent ==
  u : Inport
  A : Gain  Gain=A  Multiplication=Matrix(K*u)
  Bu : Gain  Gain=Bu  Multiplication=Matrix(K*u)
  Cy : Gain  Gain=Cy  Multiplication=Matrix(K*u)
  Integrator : Integrator  InitialCondition=x0(3*nx+1:4*nx)  ContinuousStateAttributes='x1'
  Sum5 : Sum  Inputs=|++
  y : Outport
  x : Outport  Port=2
  wires:
  Integrator/1 -> x/1, A/1, Cy/1
  A/1 -> Sum5/2
  Sum5/1 -> Integrator/1
  u/1 -> Bu/1
  Bu/1 -> Sum5/1
  Cy/1 -> y/1

== system Example_OB_Dynamic_Undirected_LeaderFollower/Agent 4/Controller ==
  "K*\\t{r(tk)}" : Inport
  "Cy*r-\\t{y}" : Inport  Port=2
  A : Gain  Gain=A  Multiplication=Matrix(K*u)
  Bu : Gain  Gain=Bu  Multiplication=Matrix(K*u)
  F : Gain  Gain=F  Multiplication=Matrix(K*u)
  Integrator : Integrator  InitialCondition=zeros(nr,1)  ContinuousStateAttributes='r1'
  Sum5 : Sum  Inputs=+++
  c : Gain  Gain=c  Multiplication=Matrix(K*u)
  r : Outport
  wires:
  A/1 -> Sum5/3
  Sum5/1 -> Integrator/1
  Integrator/1 -> r/1, A/1
  "K*\\t{r(tk)}"/1 -> c/1
  Bu/1 -> Sum5/1
  "Cy*r-\\t{y}"/1 -> F/1
  F/1 -> Sum5/2
  c/1 -> Bu/1

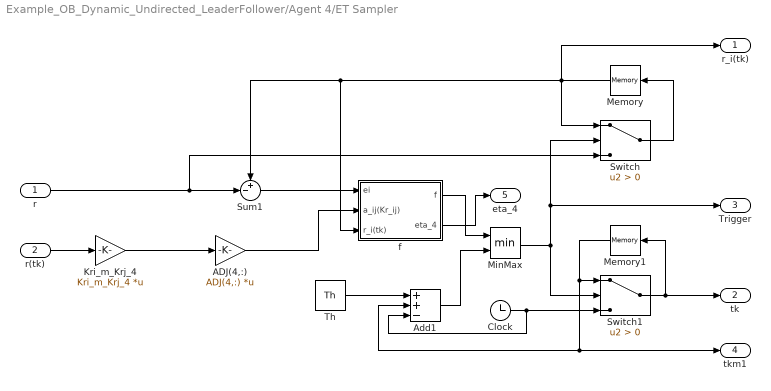
== system Example_OB_Dynamic_Undirected_LeaderFollower/Agent 4/ET Sampler ==
  r : Inport
  r(tk) : Inport  Port=2
  ADJ(4,:) : Gain  Gain=ADJ(4,:)  Multiplication=Matrix(K*u)
  Add1 : Sum  Inputs=++-
  Clock : Clock
  Kri_m_Krj_4 : Gain  Gain=Kri_m_Krj_4  Multiplication=Matrix(K*u)
  Memory : Memory  InitialCondition=zeros(nr,1)  StateName=tilde_x
  Memory1 : Memory  StateName=tilde_x
  MinMax : MinMax  Inputs=2
  Sum1 : Sum  Inputs=+-|
  Switch : Switch  Criteria=u2 > Threshold  SaturateOnIntegerOverflow=off  InputSameDT=off
  Switch1 : Switch  Criteria=u2 > Threshold  SaturateOnIntegerOverflow=off  InputSameDT=off
  Th : Constant  Value=Th
  f : Subsystem
  r_i(tk) : Outport
  tk : Outport  Port=2
  Trigger : Outport  Port=3
  tkm1 : Outport  Port=4
  eta_4 : Outport  Port=5
  wires:
  Switch1/1 -> tk/1, Memory1/1
  Switch/1 -> Memory/1
  Sum1/1 -> f/1(ei)
  r/1 -> Sum1/2, Switch/3
  Memory/1 -> r_i(tk)/1, f/3(r_i(tk)), Sum1/1, Switch/1
  r(tk)/1 -> Kri_m_Krj_4/1
  Kri_m_Krj_4/1 -> ADJ(4,:)/1
  ADJ(4,:)/1 -> f/2(a_ij(Kr_ij))
  Memory1/1 -> Switch1/1, tkm1/1, Add1/2
  Th/1 -> Add1/1
  Add1/1 -> MinMax/2
  Clock/1 -> Switch1/3, Add1/3
  f/1(f) -> MinMax/1
  MinMax/1 -> Trigger/1, Switch/2, Switch1/2
  f/2(eta_4) -> eta_4/1

== system Example_OB_Dynamic_Undirected_LeaderFollower/Agent 4/Time-triggered sampler ==
  "\\t{y}" : Inport
  Clock : Clock
  Math Function : Math  Operator=mod
  Memory : Memory  InitialCondition=ty0_4  StateName=tilde_x
  Switch : Switch  Criteria=u2 > Threshold  SaturateOnIntegerOverflow=off  InputSameDT=off
  Tc : Constant  Value=Tc(4)
  "\\t{y}(ctk)" : Outport
  wires:
  Switch/1 -> "\\t{y}(ctk)"/1, Memory/1
  "\\t{y}"/1 -> Switch/3
  Memory/1 -> Switch/1
  Tc/1 -> Math Function/2
  Clock/1 -> Math Function/1
  Math Function/1 -> Switch/2

== system Example_OB_Dynamic_Undirected_LeaderFollower/Agent 5/Agent ==
  u : Inport
  A : Gain  Gain=A  Multiplication=Matrix(K*u)
  Bu : Gain  Gain=Bu  Multiplication=Matrix(K*u)
  Cy : Gain  Gain=Cy  Multiplication=Matrix(K*u)
  Integrator : Integrator  InitialCondition=x0(4*nx+1:5*nx)  ContinuousStateAttributes='x1'
  Sum5 : Sum  Inputs=|++
  y : Outport
  x : Outport  Port=2
  wires:
  Integrator/1 -> x/1, A/1, Cy/1
  A/1 -> Sum5/2
  Sum5/1 -> Integrator/1
  u/1 -> Bu/1
  Bu/1 -> Sum5/1
  Cy/1 -> y/1

== system Example_OB_Dynamic_Undirected_LeaderFollower/Agent 5/Controller ==
  "K*\\t{r(tk)}" : Inport
  "Cy*r-\\t{y}" : Inport  Port=2
  A : Gain  Gain=A  Multiplication=Matrix(K*u)
  Bu : Gain  Gain=Bu  Multiplication=Matrix(K*u)
  F : Gain  Gain=F  Multiplication=Matrix(K*u)
  Integrator : Integrator  InitialCondition=zeros(nr,1)  ContinuousStateAttributes='r1'
  Sum5 : Sum  Inputs=+++
  c : Gain  Gain=c  Multiplication=Matrix(K*u)
  r : Outport
  wires:
  A/1 -> Sum5/3
  Sum5/1 -> Integrator/1
  Integrator/1 -> r/1, A/1
  "K*\\t{r(tk)}"/1 -> c/1
  Bu/1 -> Sum5/1
  "Cy*r-\\t{y}"/1 -> F/1
  F/1 -> Sum5/2
  c/1 -> Bu/1

== system Example_OB_Dynamic_Undirected_LeaderFollower/Agent 5/ET Sampler ==
  r : Inport
  r(tk) : Inport  Port=2
  ADJ(5,:) : Gain  Gain=ADJ(5,:)  Multiplication=Matrix(K*u)
  Add1 : Sum  Inputs=++-
  Clock : Clock
  Kri_m_Krj_5 : Gain  Gain=Kri_m_Krj_5  Multiplication=Matrix(K*u)
  Memory : Memory  InitialCondition=zeros(nr,1)  StateName=tilde_x
  Memory1 : Memory  StateName=tilde_x
  MinMax : MinMax  Inputs=2
  Sum1 : Sum  Inputs=+-|
  Switch : Switch  Criteria=u2 > Threshold  SaturateOnIntegerOverflow=off  InputSameDT=off
  Switch1 : Switch  Criteria=u2 > Threshold  SaturateOnIntegerOverflow=off  InputSameDT=off
  Th : Constant  Value=Th
  f : Subsystem
  r_i(tk) : Outport
  tk : Outport  Port=2
  Trigger : Outport  Port=3
  tkm1 : Outport  Port=4
  eta_5 : Outport  Port=5
  wires:
  Switch1/1 -> tk/1, Memory1/1
  Switch/1 -> Memory/1
  Sum1/1 -> f/1(ei)
  r/1 -> Sum1/2, Switch/3
  r(tk)/1 -> Kri_m_Krj_5/1
  Kri_m_Krj_5/1 -> ADJ(5,:)/1
  ADJ(5,:)/1 -> f/2(a_ij(Kr_ij))
  Clock/1 -> Switch1/3, Add1/3
  Th/1 -> Add1/1
  Add1/1 -> MinMax/2
  Memory1/1 -> Switch1/1, tkm1/1, Add1/2
  MinMax/1 -> Switch1/2, Switch/2, Trigger/1
  f/1(f) -> MinMax/1
  Memory/1 -> r_i(tk)/1, f/3(r_i(tk)), Sum1/1, Switch/1
  f/2(eta_5) -> eta_5/1

== system Example_OB_Dynamic_Undirected_LeaderFollower/Agent 5/Time-triggered sampler ==
  "\\t{y}" : Inport
  Clock : Clock
  Math Function : Math  Operator=mod
  Memory : Memory  InitialCondition=ty0_5  StateName=tilde_x
  Switch : Switch  Criteria=u2 > Threshold  SaturateOnIntegerOverflow=off  InputSameDT=off
  Tc : Constant  Value=Tc(5)
  "\\t{y}(ctk)" : Outport
  wires:
  Switch/1 -> "\\t{y}(ctk)"/1, Memory/1
  "\\t{y}"/1 -> Switch/3
  Memory/1 -> Switch/1
  Tc/1 -> Math Function/2
  Clock/1 -> Math Function/1
  Math Function/1 -> Switch/2

== system Example_OB_Dynamic_Undirected_LeaderFollower/Agent 6/Agent ==
  u : Inport
  A : Gain  Gain=A  Multiplication=Matrix(K*u)
  Bu : Gain  Gain=Bu  Multiplication=Matrix(K*u)
  Cy : Gain  Gain=Cy  Multiplication=Matrix(K*u)
  Integrator : Integrator  InitialCondition=x0(5*nx+1:6*nx)  ContinuousStateAttributes='x1'
  Sum5 : Sum  Inputs=|++
  y : Outport
  x : Outport  Port=2
  wires:
  Integrator/1 -> x/1, A/1, Cy/1
  A/1 -> Sum5/2
  Sum5/1 -> Integrator/1
  u/1 -> Bu/1
  Bu/1 -> Sum5/1
  Cy/1 -> y/1

== system Example_OB_Dynamic_Undirected_LeaderFollower/Agent 6/Controller ==
  "K*\\t{r(tk)}" : Inport
  "Cy*r-\\t{y}" : Inport  Port=2
  A : Gain  Gain=A  Multiplication=Matrix(K*u)
  Bu : Gain  Gain=Bu  Multiplication=Matrix(K*u)
  F : Gain  Gain=F  Multiplication=Matrix(K*u)
  Integrator : Integrator  InitialCondition=zeros(nr,1)  ContinuousStateAttributes='r1'
  Sum5 : Sum  Inputs=+++
  c : Gain  Gain=c  Multiplication=Matrix(K*u)
  r : Outport
  wires:
  A/1 -> Sum5/3
  Sum5/1 -> Integrator/1
  Integrator/1 -> r/1, A/1
  "K*\\t{r(tk)}"/1 -> c/1
  Bu/1 -> Sum5/1
  "Cy*r-\\t{y}"/1 -> F/1
  F/1 -> Sum5/2
  c/1 -> Bu/1

== system Example_OB_Dynamic_Undirected_LeaderFollower/Agent 6/ET Sampler ==
  r : Inport
  r(tk) : Inport  Port=2
  ADJ(6,:) : Gain  Gain=ADJ(6,:)  Multiplication=Matrix(K*u)
  Add1 : Sum  Inputs=++-
  Clock : Clock
  Kri_m_Krj_6 : Gain  Gain=Kri_m_Krj_6  Multiplication=Matrix(K*u)
  Memory : Memory  InitialCondition=zeros(nr,1)  StateName=tilde_x
  Memory1 : Memory  StateName=tilde_x
  MinMax : MinMax  Inputs=2
  Sum1 : Sum  Inputs=+-|
  Switch : Switch  Criteria=u2 > Threshold  SaturateOnIntegerOverflow=off  InputSameDT=off
  Switch1 : Switch  Criteria=u2 > Threshold  SaturateOnIntegerOverflow=off  InputSameDT=off
  Th : Constant  Value=Th
  f : Subsystem
  r_i(tk) : Outport
  tk : Outport  Port=2
  Trigger : Outport  Port=3
  tkm1 : Outport  Port=4
  eta_6 : Outport  Port=5
  wires:
  Switch1/1 -> tk/1, Memory1/1
  Switch/1 -> Memory/1
  Sum1/1 -> f/1(ei)
  r/1 -> Sum1/2, Switch/3
  Memory/1 -> r_i(tk)/1, f/3(r_i(tk)), Sum1/1, Switch/1
  r(tk)/1 -> Kri_m_Krj_6/1
  Kri_m_Krj_6/1 -> ADJ(6,:)/1
  ADJ(6,:)/1 -> f/2(a_ij(Kr_ij))
  Clock/1 -> Switch1/3, Add1/3
  Th/1 -> Add1/1
  Add1/1 -> MinMax/2
  Memory1/1 -> Switch1/1, Add1/2, tkm1/1
  MinMax/1 -> Switch1/2, Switch/2, Trigger/1
  f/1(f) -> MinMax/1
  f/2(eta_6) -> eta_6/1

== system Example_OB_Dynamic_Undirected_LeaderFollower/Agent 6/Time-triggered sampler ==
  "\\t{y}" : Inport
  Clock : Clock
  Math Function : Math  Operator=mod
  Memory : Memory  InitialCondition=ty0_6  StateName=tilde_x
  Switch : Switch  Criteria=u2 > Threshold  SaturateOnIntegerOverflow=off  InputSameDT=off
  Tc : Constant  Value=Tc(6)
  "\\t{y}(ctk)" : Outport
  wires:
  Switch/1 -> "\\t{y}(ctk)"/1, Memory/1
  "\\t{y}"/1 -> Switch/3
  Memory/1 -> Switch/1
  Tc/1 -> Math Function/2
  Clock/1 -> Math Function/1
  Math Function/1 -> Switch/2

== system Example_OB_Dynamic_Undirected_LeaderFollower/Agent 7/Agent ==
  u : Inport
  A : Gain  Gain=A  Multiplication=Matrix(K*u)
  Bu : Gain  Gain=Bu  Multiplication=Matrix(K*u)
  Cy : Gain  Gain=Cy  Multiplication=Matrix(K*u)
  Integrator : Integrator  InitialCondition=x0(6*nx+1:7*nx)  ContinuousStateAttributes='x1'
  Sum5 : Sum  Inputs=|++
  y : Outport
  x : Outport  Port=2
  wires:
  Integrator/1 -> x/1, A/1, Cy/1
  A/1 -> Sum5/2
  Sum5/1 -> Integrator/1
  u/1 -> Bu/1
  Bu/1 -> Sum5/1
  Cy/1 -> y/1

== system Example_OB_Dynamic_Undirected_LeaderFollower/Agent 7/Controller ==
  "K*\\t{r(tk)}" : Inport
  "Cy*r-\\t{y}" : Inport  Port=2
  A : Gain  Gain=A  Multiplication=Matrix(K*u)
  Bu : Gain  Gain=Bu  Multiplication=Matrix(K*u)
  F : Gain  Gain=F  Multiplication=Matrix(K*u)
  Integrator : Integrator  InitialCondition=zeros(nr,1)  ContinuousStateAttributes='r1'
  Sum5 : Sum  Inputs=+++
  c : Gain  Gain=c  Multiplication=Matrix(K*u)
  r : Outport
  wires:
  A/1 -> Sum5/3
  Sum5/1 -> Integrator/1
  Integrator/1 -> r/1, A/1
  "K*\\t{r(tk)}"/1 -> c/1
  Bu/1 -> Sum5/1
  "Cy*r-\\t{y}"/1 -> F/1
  F/1 -> Sum5/2
  c/1 -> Bu/1

== system Example_OB_Dynamic_Undirected_LeaderFollower/Agent 7/ET Sampler ==
  r : Inport
  r(tk) : Inport  Port=2
  ADJ(7,:) : Gain  Gain=ADJ(7,:)  Multiplication=Matrix(K*u)
  Add1 : Sum  Inputs=++-
  Clock : Clock
  Kri_m_Krj_7 : Gain  Gain=Kri_m_Krj_7  Multiplication=Matrix(K*u)
  Memory : Memory  InitialCondition=zeros(nr,1)  StateName=tilde_x
  Memory1 : Memory  StateName=tilde_x
  MinMax : MinMax  Inputs=2
  Sum1 : Sum  Inputs=+-|
  Switch : Switch  Criteria=u2 > Threshold  SaturateOnIntegerOverflow=off  InputSameDT=off
  Switch1 : Switch  Criteria=u2 > Threshold  SaturateOnIntegerOverflow=off  InputSameDT=off
  Th : Constant  Value=Th
  f : Subsystem
  r_i(tk) : Outport
  tk : Outport  Port=2
  Trigger : Outport  Port=3
  tkm1 : Outport  Port=4
  eta_7 : Outport  Port=5
  wires:
  Switch1/1 -> tk/1, Memory1/1
  Switch/1 -> Memory/1
  Sum1/1 -> f/1(ei)
  r/1 -> Sum1/2, Switch/3
  Memory/1 -> r_i(tk)/1, f/3(r_i(tk)), Sum1/1, Switch/1
  r(tk)/1 -> Kri_m_Krj_7/1
  Kri_m_Krj_7/1 -> ADJ(7,:)/1
  ADJ(7,:)/1 -> f/2(a_ij(Kr_ij))
  Clock/1 -> Switch1/3, Add1/3
  Th/1 -> Add1/1
  Add1/1 -> MinMax/2
  Memory1/1 -> Switch1/1, Add1/2, tkm1/1
  MinMax/1 -> Switch1/2, Switch/2, Trigger/1
  f/1(f) -> MinMax/1
  f/2(eta_7) -> eta_7/1

== system Example_OB_Dynamic_Undirected_LeaderFollower/Agent 7/Time-triggered sampler ==
  "\\t{y}" : Inport
  Clock : Clock
  Math Function : Math  Operator=mod
  Memory : Memory  InitialCondition=ty0_7  StateName=tilde_x
  Switch : Switch  Criteria=u2 > Threshold  SaturateOnIntegerOverflow=off  InputSameDT=off
  Tc : Constant  Value=Tc(7)
  "\\t{y}(ctk)" : Outport
  wires:
  Switch/1 -> "\\t{y}(ctk)"/1, Memory/1
  "\\t{y}"/1 -> Switch/3
  Memory/1 -> Switch/1
  Tc/1 -> Math Function/2
  Clock/1 -> Math Function/1
  Math Function/1 -> Switch/2

== system Example_OB_Dynamic_Undirected_LeaderFollower/Agent 1/ET Sampler/f ==
  ei : Inport
  a_ij(Kr_ij) : Inport  Port=2
  r_i(tk) : Inport  Port=3
  2*N*LL(1,1)+2*BB(1) : Gain  Gain=2*N*LL(1,1)+2*BB(1)  Multiplication=Matrix(K*u)
  BB(1) : Gain  Gain=BB(1)  Multiplication=Matrix(K*u)
  Dot Product1 : DotProduct  OutDataTypeStr=Inherit: Inherit via internal rule
  Dot Product2 : DotProduct  OutDataTypeStr=Inherit: Inherit via internal rule
  K : Gain  Gain=K  Multiplication=Matrix(K*u)
  K1 : Gain  Gain=K  Multiplication=Matrix(K*u)
  Sum1 : Sum  Inputs=-++
  Sum2 : Sum  Inputs=+|+
  Sum3 : Sum  Inputs=-|+
  dynamic : Subsystem
  kappa : Gain  Gain=kappa
  f : Outport
  eta_1 : Outport  Port=2
  wires:
  kappa/1 -> Sum1/3
  dynamic/1(eta) -> eta_1/1, kappa/1
  Sum3/1 -> dynamic/1(eta_u)
  Dot Product1/1 -> Sum1/2, Sum3/2
  K/1 -> Dot Product2/2, Dot Product2/1
  K1/1 -> BB(1)/1
  Dot Product2/1 -> 2*N*LL(1,1)+2*BB(1)/1
  ei/1 -> K/1
  Sum2/1 -> Dot Product1/2, Dot Product1/1
  BB(1)/1 -> Sum2/2
  a_ij(Kr_ij)/1 -> Sum2/1
  Sum1/1 -> f/1
  r_i(tk)/1 -> K1/1
  2*N*LL(1,1)+2*BB(1)/1 -> Sum3/1, Sum1/1

== system Example_OB_Dynamic_Undirected_LeaderFollower/Agent 2/ET Sampler/f ==
  ei : Inport
  a_ij(Kr_ij) : Inport  Port=2
  r_i(tk) : Inport  Port=3
  2*N*LL(2,2)+2*BB(2) : Gain  Gain=2*N*LL(2,2)+2*BB(2)  Multiplication=Matrix(K*u)
  BB(2) : Gain  Gain=BB(2)  Multiplication=Matrix(K*u)
  Dot Product1 : DotProduct  OutDataTypeStr=Inherit: Inherit via internal rule
  Dot Product2 : DotProduct  OutDataTypeStr=Inherit: Inherit via internal rule
  K : Gain  Gain=K  Multiplication=Matrix(K*u)
  K1 : Gain  Gain=K  Multiplication=Matrix(K*u)
  Sum1 : Sum  Inputs=-++
  Sum2 : Sum  Inputs=+|+
  Sum3 : Sum  Inputs=-|+
  dynamic : Subsystem
  kappa : Gain  Gain=kappa
  f : Outport
  eta_2 : Outport  Port=2
  wires:
  kappa/1 -> Sum1/3
  Sum3/1 -> dynamic/1(eta_u)
  Dot Product1/1 -> Sum1/2, Sum3/2
  K/1 -> Dot Product2/2, Dot Product2/1
  K1/1 -> BB(2)/1
  Dot Product2/1 -> 2*N*LL(2,2)+2*BB(2)/1
  ei/1 -> K/1
  Sum2/1 -> Dot Product1/2, Dot Product1/1
  BB(2)/1 -> Sum2/2
  a_ij(Kr_ij)/1 -> Sum2/1
  Sum1/1 -> f/1
  r_i(tk)/1 -> K1/1
  2*N*LL(2,2)+2*BB(2)/1 -> Sum3/1, Sum1/1
  dynamic/1(eta) -> eta_2/1, kappa/1

== system Example_OB_Dynamic_Undirected_LeaderFollower/Agent 3/ET Sampler/f ==
  ei : Inport
  a_ij(Kr_ij) : Inport  Port=2
  r_i(tk) : Inport  Port=3
  2*N*LL(3,3)+2*BB(3) : Gain  Gain=2*N*LL(3,3)+2*BB(3)  Multiplication=Matrix(K*u)
  BB(3) : Gain  Gain=BB(3)  Multiplication=Matrix(K*u)
  Dot Product1 : DotProduct  OutDataTypeStr=Inherit: Inherit via internal rule
  Dot Product2 : DotProduct  OutDataTypeStr=Inherit: Inherit via internal rule
  K : Gain  Gain=K  Multiplication=Matrix(K*u)
  K1 : Gain  Gain=K  Multiplication=Matrix(K*u)
  Sum1 : Sum  Inputs=-++
  Sum2 : Sum  Inputs=+|+
  Sum3 : Sum  Inputs=-|+
  dynamic : Subsystem
  kappa : Gain  Gain=kappa
  f : Outport
  eta_3 : Outport  Port=2
  wires:
  kappa/1 -> Sum1/3
  dynamic/1(eta) -> eta_3/1, kappa/1
  Sum3/1 -> dynamic/1(eta_u)
  Dot Product1/1 -> Sum1/2, Sum3/2
  K/1 -> Dot Product2/2, Dot Product2/1
  K1/1 -> BB(3)/1
  Dot Product2/1 -> 2*N*LL(3,3)+2*BB(3)/1
  ei/1 -> K/1
  Sum2/1 -> Dot Product1/2, Dot Product1/1
  BB(3)/1 -> Sum2/2
  a_ij(Kr_ij)/1 -> Sum2/1
  Sum1/1 -> f/1
  r_i(tk)/1 -> K1/1
  2*N*LL(3,3)+2*BB(3)/1 -> Sum3/1, Sum1/1

== system Example_OB_Dynamic_Undirected_LeaderFollower/Agent 4/ET Sampler/f ==
  ei : Inport
  a_ij(Kr_ij) : Inport  Port=2
  r_i(tk) : Inport  Port=3
  2*N*LL(4,4)+2*BB(4) : Gain  Gain=2*N*LL(4,4)+2*BB(4)  Multiplication=Matrix(K*u)
  BB(4) : Gain  Gain=BB(4)  Multiplication=Matrix(K*u)
  Dot Product1 : DotProduct  OutDataTypeStr=Inherit: Inherit via internal rule
  Dot Product2 : DotProduct  OutDataTypeStr=Inherit: Inherit via internal rule
  K : Gain  Gain=K  Multiplication=Matrix(K*u)
  K1 : Gain  Gain=K  Multiplication=Matrix(K*u)
  Sum1 : Sum  Inputs=-++
  Sum2 : Sum  Inputs=+|+
  Sum3 : Sum  Inputs=-|+
  dynamic : Subsystem
  kappa : Gain  Gain=kappa
  f : Outport
  eta_4 : Outport  Port=2
  wires:
  kappa/1 -> Sum1/3
  dynamic/1(eta) -> eta_4/1, kappa/1
  Sum3/1 -> dynamic/1(eta_u)
  Dot Product1/1 -> Sum1/2, Sum3/2
  K/1 -> Dot Product2/2, Dot Product2/1
  K1/1 -> BB(4)/1
  Dot Product2/1 -> 2*N*LL(4,4)+2*BB(4)/1
  ei/1 -> K/1
  Sum2/1 -> Dot Product1/2, Dot Product1/1
  BB(4)/1 -> Sum2/2
  a_ij(Kr_ij)/1 -> Sum2/1
  Sum1/1 -> f/1
  r_i(tk)/1 -> K1/1
  2*N*LL(4,4)+2*BB(4)/1 -> Sum3/1, Sum1/1

== system Example_OB_Dynamic_Undirected_LeaderFollower/Agent 5/ET Sampler/f ==
  ei : Inport
  a_ij(Kr_ij) : Inport  Port=2
  r_i(tk) : Inport  Port=3
  2*N*LL(5,5)+2*BB(5) : Gain  Gain=2*N*LL(5,5)+2*BB(5)  Multiplication=Matrix(K*u)
  BB(5) : Gain  Gain=BB(5)  Multiplication=Matrix(K*u)
  Dot Product1 : DotProduct  OutDataTypeStr=Inherit: Inherit via internal rule
  Dot Product2 : DotProduct  OutDataTypeStr=Inherit: Inherit via internal rule
  K : Gain  Gain=K  Multiplication=Matrix(K*u)
  K1 : Gain  Gain=K  Multiplication=Matrix(K*u)
  Sum1 : Sum  Inputs=-++
  Sum2 : Sum  Inputs=+|+
  Sum3 : Sum  Inputs=-|+
  dynamic : Subsystem
  kappa : Gain  Gain=kappa
  f : Outport
  eta_5 : Outport  Port=2
  wires:
  kappa/1 -> Sum1/3
  dynamic/1(eta) -> eta_5/1, kappa/1
  Sum3/1 -> dynamic/1(eta_u)
  Dot Product1/1 -> Sum1/2, Sum3/2
  K/1 -> Dot Product2/2, Dot Product2/1
  K1/1 -> BB(5)/1
  Dot Product2/1 -> 2*N*LL(5,5)+2*BB(5)/1
  ei/1 -> K/1
  Sum2/1 -> Dot Product1/2, Dot Product1/1
  BB(5)/1 -> Sum2/2
  a_ij(Kr_ij)/1 -> Sum2/1
  Sum1/1 -> f/1
  r_i(tk)/1 -> K1/1
  2*N*LL(5,5)+2*BB(5)/1 -> Sum3/1, Sum1/1

== system Example_OB_Dynamic_Undirected_LeaderFollower/Agent 6/ET Sampler/f ==
  ei : Inport
  a_ij(Kr_ij) : Inport  Port=2
  r_i(tk) : Inport  Port=3
  2*N*LL(6,6)+2*BB(6) : Gain  Gain=2*N*LL(6,6)+2*BB(6)  Multiplication=Matrix(K*u)
  BB(6) : Gain  Gain=BB(6)  Multiplication=Matrix(K*u)
  Dot Product1 : DotProduct  OutDataTypeStr=Inherit: Inherit via internal rule
  Dot Product2 : DotProduct  OutDataTypeStr=Inherit: Inherit via internal rule
  K : Gain  Gain=K  Multiplication=Matrix(K*u)
  K1 : Gain  Gain=K  Multiplication=Matrix(K*u)
  Sum1 : Sum  Inputs=-++
  Sum2 : Sum  Inputs=+|+
  Sum3 : Sum  Inputs=-|+
  dynamic : Subsystem
  kappa : Gain  Gain=kappa
  f : Outport
  eta_6 : Outport  Port=2
  wires:
  kappa/1 -> Sum1/3
  dynamic/1(eta) -> eta_6/1, kappa/1
  Sum3/1 -> dynamic/1(eta_u)
  Dot Product1/1 -> Sum1/2, Sum3/2
  K/1 -> Dot Product2/2, Dot Product2/1
  K1/1 -> BB(6)/1
  Dot Product2/1 -> 2*N*LL(6,6)+2*BB(6)/1
  ei/1 -> K/1
  Sum2/1 -> Dot Product1/2, Dot Product1/1
  BB(6)/1 -> Sum2/2
  a_ij(Kr_ij)/1 -> Sum2/1
  Sum1/1 -> f/1
  r_i(tk)/1 -> K1/1
  2*N*LL(6,6)+2*BB(6)/1 -> Sum3/1, Sum1/1

== system Example_OB_Dynamic_Undirected_LeaderFollower/Agent 7/ET Sampler/f ==
  ei : Inport
  a_ij(Kr_ij) : Inport  Port=2
  r_i(tk) : Inport  Port=3
  2*N*LL(7,7)+2*BB(7) : Gain  Gain=2*N*LL(7,7)+2*BB(7)  Multiplication=Matrix(K*u)
  BB(7) : Gain  Gain=BB(7)  Multiplication=Matrix(K*u)
  Dot Product1 : DotProduct  OutDataTypeStr=Inherit: Inherit via internal rule
  Dot Product2 : DotProduct  OutDataTypeStr=Inherit: Inherit via internal rule
  K : Gain  Gain=K  Multiplication=Matrix(K*u)
  K1 : Gain  Gain=K  Multiplication=Matrix(K*u)
  Sum1 : Sum  Inputs=-++
  Sum2 : Sum  Inputs=+|+
  Sum3 : Sum  Inputs=-|+
  dynamic : Subsystem
  kappa : Gain  Gain=kappa
  f : Outport
  eta_7 : Outport  Port=2
  wires:
  ei/1 -> K/1
  K/1 -> Dot Product2/2, Dot Product2/1
  Sum1/1 -> f/1
  Dot Product2/1 -> 2*N*LL(7,7)+2*BB(7)/1
  a_ij(Kr_ij)/1 -> Sum2/1
  2*N*LL(7,7)+2*BB(7)/1 -> Sum3/1, Sum1/1
  K1/1 -> BB(7)/1
  r_i(tk)/1 -> K1/1
  BB(7)/1 -> Sum2/2
  Sum2/1 -> Dot Product1/2, Dot Product1/1
  Dot Product1/1 -> Sum1/2, Sum3/2
  Sum3/1 -> dynamic/1(eta_u)
  dynamic/1(eta) -> eta_7/1, kappa/1
  kappa/1 -> Sum1/3

== system Example_OB_Dynamic_Undirected_LeaderFollower/Agent 1/ET Sampler/f/dynamic ==
  eta_u : Inport
  A : Gain  Gain=-delta
  Integrator : Integrator  InitialCondition=eta1  ContinuousStateAttributes='eta1'
  Sum5 : Sum  Inputs=|++
  mu : Gain  Gain=mu
  eta : Outport
  wires:
  Integrator/1 -> A/1, eta/1
  A/1 -> Sum5/2
  Sum5/1 -> Integrator/1
  eta_u/1 -> mu/1
  mu/1 -> Sum5/1

== system Example_OB_Dynamic_Undirected_LeaderFollower/Agent 2/ET Sampler/f/dynamic ==
  eta_u : Inport
  A : Gain  Gain=-delta
  Integrator : Integrator  InitialCondition=eta2  ContinuousStateAttributes='eta2'
  Sum5 : Sum  Inputs=|++
  mu : Gain  Gain=mu
  eta : Outport
  wires:
  Integrator/1 -> A/1, eta/1
  A/1 -> Sum5/2
  Sum5/1 -> Integrator/1
  eta_u/1 -> mu/1
  mu/1 -> Sum5/1

== system Example_OB_Dynamic_Undirected_LeaderFollower/Agent 3/ET Sampler/f/dynamic ==
  eta_u : Inport
  A : Gain  Gain=-delta
  Integrator : Integrator  InitialCondition=eta3  ContinuousStateAttributes='eta3'
  Sum5 : Sum  Inputs=|++
  mu : Gain  Gain=mu
  eta : Outport
  wires:
  Integrator/1 -> A/1, eta/1
  A/1 -> Sum5/2
  Sum5/1 -> Integrator/1
  eta_u/1 -> mu/1
  mu/1 -> Sum5/1

== system Example_OB_Dynamic_Undirected_LeaderFollower/Agent 4/ET Sampler/f/dynamic ==
  eta_u : Inport
  A : Gain  Gain=-delta
  Integrator : Integrator  InitialCondition=eta4  ContinuousStateAttributes='eta4'
  Sum5 : Sum  Inputs=|++
  mu : Gain  Gain=mu
  eta : Outport
  wires:
  Integrator/1 -> A/1, eta/1
  A/1 -> Sum5/2
  Sum5/1 -> Integrator/1
  eta_u/1 -> mu/1
  mu/1 -> Sum5/1

== system Example_OB_Dynamic_Undirected_LeaderFollower/Agent 5/ET Sampler/f/dynamic ==
  eta_u : Inport
  A : Gain  Gain=-delta
  Integrator : Integrator  InitialCondition=eta5  ContinuousStateAttributes='eta5'
  Sum5 : Sum  Inputs=|++
  mu : Gain  Gain=mu
  eta : Outport
  wires:
  Integrator/1 -> A/1, eta/1
  A/1 -> Sum5/2
  Sum5/1 -> Integrator/1
  eta_u/1 -> mu/1
  mu/1 -> Sum5/1

== system Example_OB_Dynamic_Undirected_LeaderFollower/Agent 6/ET Sampler/f/dynamic ==
  eta_u : Inport
  A : Gain  Gain=-delta
  Integrator : Integrator  InitialCondition=eta6  ContinuousStateAttributes='eta6'
  Sum5 : Sum  Inputs=|++
  mu : Gain  Gain=mu
  eta : Outport
  wires:
  Integrator/1 -> A/1, eta/1
  A/1 -> Sum5/2
  Sum5/1 -> Integrator/1
  eta_u/1 -> mu/1
  mu/1 -> Sum5/1

== system Example_OB_Dynamic_Undirected_LeaderFollower/Agent 7/ET Sampler/f/dynamic ==
  eta_u : Inport
  A : Gain  Gain=-delta
  Integrator : Integrator  InitialCondition=eta1  ContinuousStateAttributes='eta1'
  Sum5 : Sum  Inputs=|++
  mu : Gain  Gain=mu
  eta : Outport
  wires:
  Integrator/1 -> A/1, eta/1
  A/1 -> Sum5/2
  Sum5/1 -> Integrator/1
  eta_u/1 -> mu/1
  mu/1 -> Sum5/1
